simulink model "send"  (R2024b)
settings: Solver=FixedStepAuto  StartTime=0.0  StopTime=10.0  FixedStep=0.02  RelTol=1e-3
settings Model: Creator=Amin  LastModifiedBy=Amin
settings OptimizationCC: DefaultParameterBehavior=Inlined  EnhancedBackFolding=on  PassReuseOutputArgsAs=Individual arguments  ZeroExternalMemoryAtStartup=off  ZeroInternalMemoryAtStartup=off  OptimizeBlockOrder=speed  DifferentSizesBufferReuse=on  OptimizationCustomize=off  EfficientTunableParamExpr=on
settings DebuggingCC: ParameterTunabilityLossMsg=error
settings SFSimCC: MATLABDynamicMemAlloc=off
settings RTWCC: Description=Embedded Coder  SystemTargetFile=ert.tlc  GenCodeOnly=on  TemplateMakefile=ert_default_tmf  CustomSourceCode=extern QQueue<uint8_t> globalQueue;  DataTypeReplacement=CDataTypesFixedWidth  TargetLang=C++
settings RTWCC: CustomHeaderCode=|
  | #include <QQueue>
  | #include <QDebug>
settings CodeAppCC: ForceParamTrailComments=on  IgnoreCustomStorageClasses=off  OperatorAnnotations=on  SimulinkDataObjDesc=on  SFDataObjDesc=on  InsertBlockDesc=on
settings ERTTargetCC: TargetLangStandard=C++11 (ISO)  GenerateSampleERTMain=on  CodeInterfacePackaging=C++ class  SupportComplex=off  ParenthesesLevel=Minimum  RootIOFormat=Structure reference  ERTCustomFileTemplate=example_file_process.tlc  ERTFilePackagingFormat=Compact  MaxIdInt64=INT64_MAX  MinIdInt64=INT64_MIN  MaxIdUint64=UINT64_MAX  MaxIdInt32=INT32_MAX  MinIdInt32=INT32_MIN  MaxIdUint32=UINT32_MAX  MaxIdInt16=INT16_MAX  MinIdInt16=INT16_MIN  MaxIdUint16=UINT16_MAX  MaxIdInt8=INT8_MAX  MinIdInt8=INT8_MIN  MaxIdUint8=UINT8_MAX

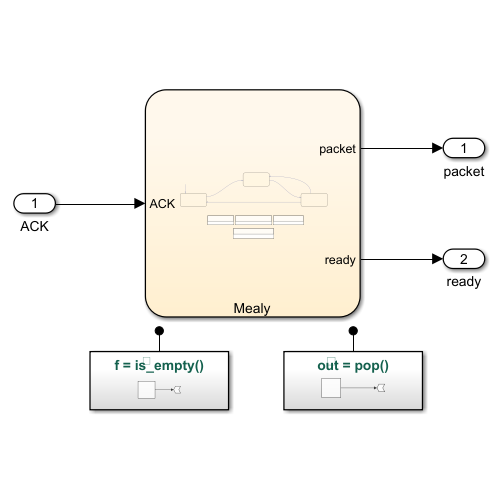
[thumbnail: Simulink's stored preview of the top-level diagram]
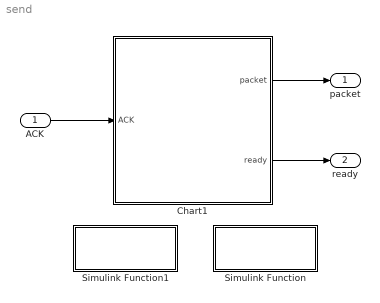
== system send ==
  ACK : Inport
  Chart1 : Stateflow chart  TreatAsAtomicUnit=on
  Simulink Function : Subsystem  TreatAsAtomicUnit=on
  Simulink Function1 : Subsystem  TreatAsAtomicUnit=on
  packet : Outport
  ready : Outport  Port=2
  wires:
  ACK/1 -> Chart1/1(ACK)
  Chart1/1(packet) -> packet/1
  Chart1/2(ready) -> ready/1

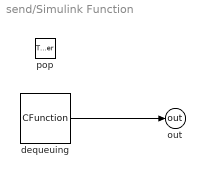
== system send/Simulink Function ==
  pop : TriggerPort  TriggerType=function-call  IsSimulinkFunction=on  FunctionName=pop  FunctionVisibility=scoped  VariantControl=(inherit)
  dequeuing : CFunction  OutputCode=out = globalQueue.dequeue();  CodegenOutputCode=out = globalQueue.dequeue();
  out : ArgOut  OutDataTypeStr=uint8  ArgumentName=out
  wires:
  dequeuing/1 -> out/1

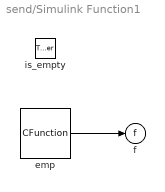
== system send/Simulink Function1 ==
  is_empty : TriggerPort  TriggerType=function-call  IsSimulinkFunction=on  FunctionName=is_empty  FunctionVisibility=scoped  VariantControl=(inherit)
  emp : CFunction  OutputCode=|  CodegenOutputCode=|
      OutputCode=|
      | if (globalQueue.isEmpty())
      |     flag = true;
      | else
      |     flag = false;
      CodegenOutputCode=|
      | if (globalQueue.isEmpty())
      |     flag = true;
      | else
      |     flag = false;
  f : ArgOut  OutDataTypeStr=boolean  ArgumentName=f
  wires:
  emp/1 -> f/1

== stateflow chart send/Chart1 ==
  settings: stateMachineType=MEALY_MACHINE  executeAtInitialization=1
  state Send_packet
  state Idle
  state Wait_for_ack
  Idle -> Send_packet : [~is_empty()]{data = pop(); packet = uint16(calculation(data, tag)); ready = true;}
  Wait_for_ack -> Send_packet [order 2] : [after(TIMEOUT, sec)]{packet = uint16(calculation(data, tag)); ready = true;}
  Send_packet -> Wait_for_ack [order 2] : {ready = false;}
  Send_packet -> Idle [order 1] : [checkACK(ACK, c_ACK)]
      | {c_ACK = reset_ACK(c_ACK); tag = 1-tag; ready = false;}
  (default) -> Idle
  Wait_for_ack -> Idle [order 1] : [checkACK(ACK, c_ACK)]{c_ACK = reset_ACK(c_ACK); tag = 1-tag;}
  data: f function_output; ack function_input; check function_input; value function_input; t function_input; header function_output; polynomial function_input; input function_input uint8; output function_output uint16; c_tag function_input; value function_input; header function_output; polynomial function_input; ca function_input; new_ca function_output; TIMEOUT constant double =4; packet output uint16; ACK input uint8; c_ACK local uint8 =1; tag local single =1; data local uint8 =0; ready output boolean
  function f = checkACK(ack, check):
    | function f = checkACK(ack, check)
    | 
    |     header = uint8(bitshift(ack, -4));
    |     ack_value = uint8(bitand(ack, 0x0F));
    |     if ack_crc(ack_value, 19) == header && ack_value == check
    |         f = true;
    |     else
    |         f = false;
    |     end
    |     
    | end
  function header = crc4(value, t, polynomial):
    | function header = crc4(value, t, polynomial)
    |         
    |     % Initialize the CRC register to 0
    |     crc = uint16(0);
    |     input = bitor(uint16(value), bitshift(uint16(t), 8));
    |         
    |     % Loop over each bit in the input byte (MSB first)
    |     for i = 8:-1:-4
    |         % XOR the MSB of the input with the MSB of the CRC register
    |         crc = bitxor(crc, bitand(bitshift(input, -i), 1));  % Shift input and XOR
    |             
    |         % If the MSB of the CRC is 1, perform the polynomial division (XOR)
    |         if bitget(crc, 5)  % Check if MSB (bit 5) of 8-bit crc is set
    |            crc = bitxor(crc, polynomial);  % Perform division by XOR with polynomial
    |         end
    |             
    |         if i ~= -4
    |             % Shift CRC register left by 1 bit
    |             crc = bitshift(crc, 1);
    |         end
    |     end
    |         
    |     
    |     % Final CRC value is the remainder in the lowest 4 bits
    |     header = uint8(bitand(crc, 15));  % Mask to get the lower 4 bits as the CRC result
    | end
  function output = calculation(input, c_tag):
    | function output = calculation(input, c_tag)
    |     
    |     
    |     output = bitor(bitor(uint16(input), bitshift(uint16(c_tag), 8)), bitshift(uint16(crc4(input, c_tag, 19)), 9));
    | 
    | end
  function header = ack_crc(value, polynomial):
    | function header = ack_crc(value, polynomial)
    |         
    |     % Initialize the CRC register to 0
    |     crc = uint8(0);
    |         
    |     % Loop over each bit in the input byte (MSB first)
    |     for i = 7:-1:-4
    |         % XOR the MSB of the input with the MSB of the CRC register
    |         crc = bitxor(crc, bitand(bitshift(value, -i), 1));  % Shift input and XOR
    |             
    |         % If the MSB of the CRC is 1, perform the polynomial division (XOR)
    |         if bitget(crc, 5)  % Check if MSB (bit 5) of 8-bit crc is set
    |            crc = bitxor(crc, polynomial);  % Perform division by XOR with polynomial
    |         end
    |             
    |         if i ~= -4
    |             % Shift CRC register left by 1 bit
    |             crc = bitshift(crc, 1);
    |         end
    |     end
    |         
    |     
    |     % Final CRC value is the remainder in the lowest 4 bits
    |     header = bitand(crc, 15);  % Mask to get the lower 4 bits as the CRC result
    | end
  function new_ca = reset_ACK(ca):
    | function new_ca = reset_ACK(ca)
    | 
    |     if ca == 255
    |         new_ca = uint8(0);
    |     else
    |         new_ca = uint8(ca + 1);
    |     end
    | end
